simulink model "geo_affine"  (Simulink 10.1)
settings: Solver=FixedStepDiscrete  StartTime=0.0  StopTime=0  RelTol=1e-3  EnableMultiTasking=on
undefined symbols (not defined in the file or in its folder): gray
libraries: vipobslib x1, visionsources x1, visiongeotforms x1
settings Model: Creator=FxMain  LastModifiedBy=panos
settings DataIOCC: LimitDataPoints=on  SignalLoggingSaveFormat=ModelDataLogs
settings OptimizationCC: ExpressionDepthLimit=2147483647
settings DebuggingCC: SolverPrmCheckMsg=warning  FcnCallInpInsideContextMsg=warning  StateNameClashWarn=warning
settings ConfigComp: CovExternalEMLEnable=on

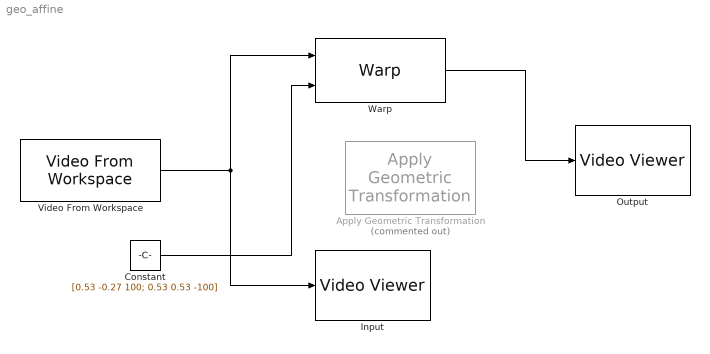
== system geo_affine ==
  Apply Geometric Transformation : vipobslib/Apply Geometric Transformation  Commented=on  tformSource=Input port  tformValue=[1 0 0; 0 1 0; 0 0 1]  approxProjectiveFlag=off  errorTolerance=1.0  roiMethod=Whole input image  roiSource=Input port  roiBBox=[0 0 128 256]  roiVertice=[0 0 10 12 20 22]  inputClipFlag=off  interpolationMethod=Bilinear  fillValue=0  viewPortMethod=Same as input image  outputSize=[512 512]  outputLoc=[0 0]  outputClipFlag=off
      settings: SourceProductBaseCode=VP
  Constant : Constant  Value=[0.53 -0.27 100; 0.53 0.53 -100]  VectorParams1D=off
      settings: SamplingMode=Frame based
  Input : VideoViewer  colormapValue=gray(256)  FigPos=[271 1025 838 674]
  Output : VideoViewer  colormapValue=gray(256)  FigPos=[1027 876 628 558]
  Video From Workspace : visionsources/Video From Workspace  signal=img  Ts=1  finalout=Obsolete  finaloutActive=Cyclic repetition  imagePorts=One multidimensional signal  OutPortLabels=R|G|B
      settings: SourceProductBaseCode=VP
  Warp : visiongeotforms/Warp  TransformMatrixSource=Input port  TransformMatrix=eye( 3 )  InterpolationMethod=Bilinear  BackgroundFillValue=0  OutputImagePositionSource=Same as input image  OutputImagePosition=[ 1, 1, 512, 512 ]  ROIInputPort=off  ROIValidityOutputPort=off  SimulateUsing=Interpreted execution
      settings: SourceProductBaseCode=VP
  wires:
  Video From Workspace/1 -> Warp/1, Input/1
  Warp/1 -> Output/1
  Constant/1 -> Warp/2
